simulink model "rct_powerstage"  (R2022a)
settings: Solver=FixedStepDiscrete  StartTime=0.0  StopTime=2e-4  RelTol=1e-3  EnableMultiTasking=on
PreLoadFcn:
  | load PowerStageData
undefined symbols (not defined in the file or in its folder): Tm, Vmax
libraries: cstblocks x1
settings Model: Creator=The MathWorks, Inc.  LastModifiedBy=The MathWorks, Inc.
settings SolverCC: AlgebraicLoopSolver=TrustRegion  MaxZcPerStep=1
settings DataIOCC: LimitDataPoints=on  SaveFormat=Array  SaveOutput=off  SaveTime=off  ReturnWorkspaceOutputs=off
settings OptimizationCC: ExpressionDepthLimit=2147483647  InitFltsAndDblsToZero=on  LifeSpan=inf
settings DebuggingCC: SaveWithParameterizedLinksMsg=none  UnderspecifiedInitializationDetection=Classic  MergeDetectMultiDrivingBlocksExec=none  SignalResolutionControl=TryResolveAllWithWarning  SolverPrmCheckMsg=warning  MultiTaskDSMMsg=warning  MultiTaskCondExecSysMsg=none  FcnCallInpInsideContextMsg=warning  UnconnectedInputMsg=warning  UnconnectedOutputMsg=warning  UnconnectedLineMsg=warning  StateNameClashWarn=warning  SFUnexpectedBacktrackingDiag=warning  SFNoUnconditionalDefaultTransitionDiag=warning  SFExecutionAtInitializationDiag=none  SFMachineParentedDataDiag=warning  ArithmeticOperatorsInVariantConditions=warning
settings HardwareCC: ProdBitPerPointer=32  ProdBitPerSizeT=32  ProdBitPerPtrDiffT=32  ProdLargestAtomicFloat=None  ProdIntDivRoundTo=Undefined  ProdEndianess=Unspecified  ProdWordSize=32  ProdHWDeviceType=32-bit Generic
settings ModelReferenceCC: PropagateSignalLabelsOutOfModel=off
settings SFSimCC: SimUseLocalCustomCode=off  SimParseCustomCode=off  CustomCodeUndefinedFunction=UseInterfaceOnly
settings RTWCC: RTWUseLocalCustomCode=off  DLArmComputeVersion=19.05
settings CodeAppCC: StateflowObjectComments=on
settings GRTTargetCC: TargetFcnLib=ansi_tfl_tmw.mat  TargetLangStandard=C89/C90 (ANSI)  CombineOutputUpdateFcns=off  GRTInterface=on
settings ConfigComp: CovMetricSettings=dw  CovSaveCumulativeToWorkspaceVar=on  CovSaveSingleToWorkspaceVar=on  CovExternalEMLEnable=off

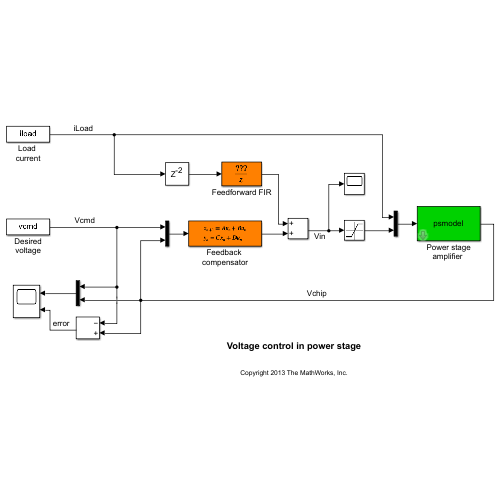
[thumbnail: Simulink's stored preview of the top-level diagram]
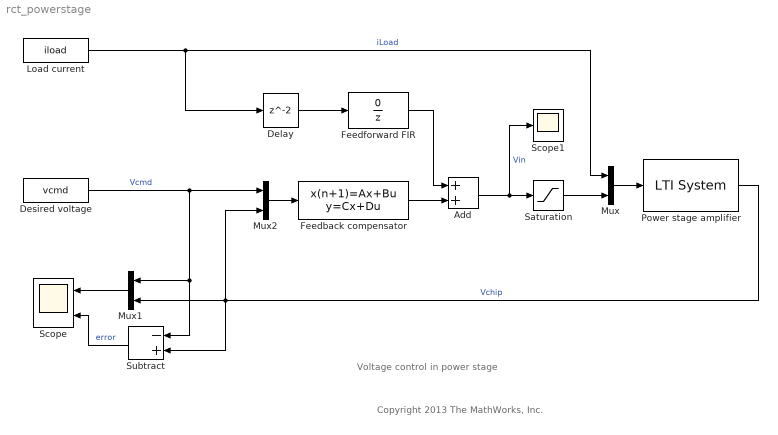
== system rct_powerstage ==
  note: Copyright 2013 The MathWorks, Inc.
  note: Voltage control in power stage
  Add : Sum
  Delay : Delay  SampleTime=Tm
  Desired voltage : FromWorkspace  VariableName=vcmd  SampleTime=Tm
  Feedback compensator : DiscreteStateSpace  A=0.5*eye(3)  B=ones(3,2)  C=ones(1,3)  D=[0 0]  SampleTime=Tm
  Feedforward FIR : DiscreteTransferFcn  Numerator=[0 0]  Denominator=[1 0]  SampleTime=Tm
  Load current : FromWorkspace  VariableName=iload  SampleTime=Tm
  Mux : Mux  Inputs=2
  Mux1 : Mux  Inputs=2
  Mux2 : Mux  Inputs=2
  "Power stage amplifier " : cstblocks/LTI System  sys=psmodel  IC=[]
  Saturation : Saturate  UpperLimit=Vmax  LowerLimit=-Vmax
  Scope : Scope  NumInputPorts=2
  Scope1 : Scope
  Subtract : Sum  Inputs=-+
  wires:
  Load current/1 -> Mux/1, Delay/1  "iLoad"
  Delay/1 -> Feedforward FIR/1
  Mux2/1 -> Feedback compensator/1
  Add/1 -> Saturation/1, Scope1/1  "Vin"
  "Power stage amplifier "/1 -> Subtract/2, Mux2/2, Mux1/2  "Vchip"
  Mux/1 -> "Power stage amplifier "/1
  Desired voltage/1 -> Subtract/1, Mux1/1, Mux2/1  "Vcmd"
  Feedforward FIR/1 -> Add/1
  Mux1/1 -> Scope/1
  Subtract/1 -> Scope/2  "error"
  Feedback compensator/1 -> Add/2
  Saturation/1 -> Mux/2
